simulink model "Quinto"  (R2017b)
settings: Solver=VariableStepAuto  StartTime=0.0  StopTime=5  RelTol=1e-3
settings Model: Creator=Cx001la  LastModifiedBy=Cx001la

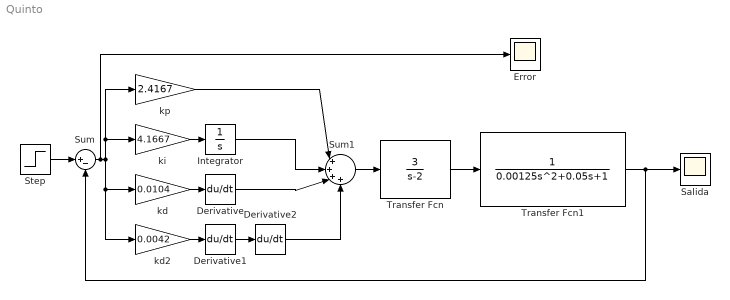
== system Quinto ==
  Derivative : Derivative
  Derivative1 : Derivative
  Derivative2 : Derivative
  Error : Scope
  Integrator : Integrator
  Salida : Scope
  Step : Step  Time=0  SampleTime=0
  Sum : Sum  Inputs=|+-
  Sum1 : Sum  Inputs=|++++
  Transfer Fcn : TransferFcn  Numerator=[3]  Denominator=[1 -2]
  Transfer Fcn1 : TransferFcn  Denominator=[0.00125 0.05 1]
  kd : Gain  Gain=0.0104
  kd2 : Gain  Gain=0.0042
  ki : Gain  Gain=4.1667
  kp : Gain  Gain=2.4167
  wires:
  Step/1 -> Sum/1
  Sum/1 -> Error/1, kp/1, ki/1, kd2/1, kd/1
  ki/1 -> Integrator/1
  kd/1 -> Derivative/1
  kd2/1 -> Derivative1/1
  Derivative1/1 -> Derivative2/1
  Derivative2/1 -> Sum1/4
  Derivative/1 -> Sum1/3
  Integrator/1 -> Sum1/2
  kp/1 -> Sum1/1
  Sum1/1 -> Transfer Fcn/1
  Transfer Fcn/1 -> Transfer Fcn1/1
  Transfer Fcn1/1 -> Salida/1, Sum/2
